simulink model "iddemo_cstr"  (R2016a)
settings: Solver=ode45  StartTime=0  StopTime=800  MaxStep=0.2  RelTol=1e-3
model workspace (MATLAB code in the model file):
  | %Model constants
  | k0                = 34930800;
  | DeltaER       = 5963.6;
  | DeltaH         = -11.92;
  | UA               = 0.3;
  | FV_plus_UA = 1.3;
  | 
  | %Fixed IC
  | Concentration0 = 1.5;
  | FeedCon0         = 10;
  | FeedTemp0       = 295;
  | 
  | %Derived IC
  | tmpVal = FeedCon0/Concentration0-1;
  | ReactorTemp0 = -DeltaER/log(tmpVal/k0);
  | CoolantTemp0 = (ReactorTemp0*(FV_plus_UA)+tmpVal*Concentration0*DeltaH-FeedTemp0)/UA;
  | 
  | %
  | tStep = 400; % [s] When the step reference change happens
  | Ts = 0.1; % [s] Sample time
  | 
  | % Scaling factors on the signals
  | CAscale = 10;
  | Tjscale = 1/10;
  | 
  | % Moving average filter
  | N = 100;
  | 
  | %Clean up
  | clear tmpVal
undefined symbols (not defined in the file or in its folder): sigbuilder_block
libraries: simulink x3, slident x1
settings Model: Creator=The MathWorks, Inc.  LastModifiedBy=The MathWorks, Inc.
settings DataIOCC: InitialState=[311.267; 8.5695]  SaveFormat=Array  SaveOutput=off  SignalLogging=off  DSMLogging=off  SaveTime=off  SignalLoggingName=logsOut
settings OptimizationCC: BlockReduction=off  BooleanDataType=off  DefaultParameterBehavior=Inlined  InlineInvariantSignals=on  BufferReuse=off  ExpressionDepthLimit=2147483647  InitFltsAndDblsToZero=on
settings DebuggingCC: SaveWithParameterizedLinksMsg=none  UnderspecifiedInitializationDetection=Classic  MergeDetectMultiDrivingBlocksExec=none  CheckExecutionContextPreStartOutputMsg=on  CheckExecutionContextRuntimeOutputMsg=on  SignalResolutionControl=TryResolveAllWithWarning  MultiTaskDSMMsg=warning  MultiTaskCondExecSysMsg=none  FcnCallInpInsideContextMsg=UseLocalSettings  AllowSymbolicDim=off  StateNameClashWarn=warning
settings HardwareCC: ProdBitPerPointer=32  ProdLargestAtomicFloat=None  ProdIntDivRoundTo=Undefined  ProdEndianess=Unspecified  ProdWordSize=32  ProdHWDeviceType=32-bit Generic  TargetUnknown=on
settings ModelReferenceCC: PropagateSignalLabelsOutOfModel=off
settings GRTTargetCC: TargetFcnLib=ansi_tfl_tmw.mat  CombineOutputUpdateFcns=off  GRTInterface=on
settings ConfigComp: CovModelRefEnable=Off  CovSFcnEnable=off

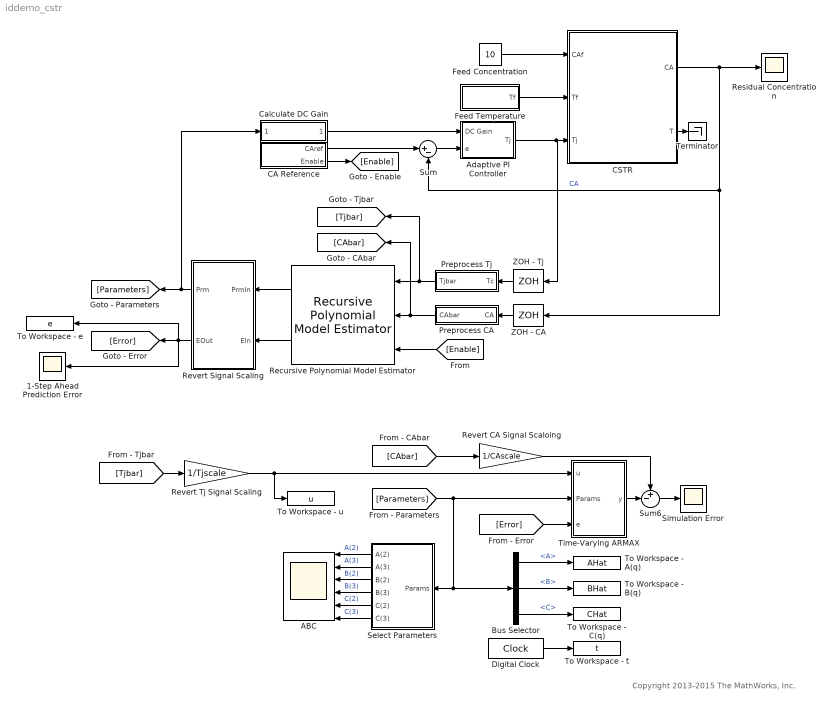
== system iddemo_cstr ==
  note: Copyright 2013-2015 The MathWorks, Inc.
  " Revert CA Signal Scaloing" : Gain  Gain=1/CAscale
  1-Step Ahead Prediction Error : Scope
  ABC : Scope  NumInputPorts=6
  Adaptive PI Controller : Subsystem
  Bus Selector : BusSelector  OutputSignals=A,B,C
  CA Reference : Subsystem
  CSTR : Subsystem
  Calculate DC Gain : Subsystem
  Digital Clock : DigitalClock  SampleTime=Ts
  Feed Concentration : Constant  Value=10
  Feed Temperature : Subsystem
  Preprocess CA : Subsystem
  Preprocess Tj : Subsystem
  Recursive Polynomial Model Estimator : slident/Estimators/Recursive Polynomial Model Estimator  ModelStructure=ARMAX  InitialEstimateSource=None  A0=2  B0=2  C0=2  D0=1  F0=1  nk=1  P0=1e4  EstimationMethod=Forgetting Factor  AdaptationParameter=1-5e-3  NormalizationBias=eps  OutputError=on  OutputP=off  AddEnablePort=on  Ts=0.1
  Residual Concentration : Scope
  Revert Signal Scaling : Subsystem
  Revert Tj Signal Scaling : Gain  Gain=1/Tjscale
  Select Parameters : Subsystem
  Simulation Error : Scope
  Sum : Sum  Inputs=|+-
  Sum6 : Sum  Inputs=+-|
  Terminator : Terminator
  Time-Varying ARMAX : Subsystem
  To Workspace - A(q) : ToWorkspace  VariableName=AHat  SampleTime=-1
  To Workspace - B(q) : ToWorkspace  VariableName=BHat  SampleTime=-1
  To Workspace - C(q) : ToWorkspace  VariableName=CHat  SampleTime=-1
  To Workspace - e : ToWorkspace  VariableName=e  SampleTime=-1
  To Workspace - t : ToWorkspace  VariableName=t  SampleTime=-1
  To Workspace - u : ToWorkspace  VariableName=u  SampleTime=-1
  ZOH - CA : ZeroOrderHold  SampleTime=Ts
  ZOH - Tj : ZeroOrderHold  SampleTime=Ts
  wires:
  CSTR/2(T) -> Terminator/1
  Preprocess Tj/1(Tjbar) -> Recursive Polynomial Model Estimator/1, [Tjbar]
  Preprocess CA/1(CAbar) -> Recursive Polynomial Model Estimator/2, [CAbar]
  Recursive Polynomial Model Estimator/1 -> Revert Signal Scaling/1(PrmIn)
  CSTR/1(CA) -> Residual Concentration/1, ZOH - CA/1, Sum/2  "CA"
  Feed Concentration/1 -> CSTR/1(CAf)
  CA Reference/1(CAref) -> Sum/1
  Feed Temperature/1(Tf) -> CSTR/2(Tf)
  CA Reference/2(Enable) -> [Enable]
  [Enable] -> Recursive Polynomial Model Estimator/3
  Recursive Polynomial Model Estimator/2 -> Revert Signal Scaling/2(EIn)
  Revert Signal Scaling/1(Prm) -> [Parameters], Calculate DC Gain/1(Params)
  ZOH - Tj/1 -> Preprocess Tj/1(Tc)
  ZOH - CA/1 -> Preprocess CA/1(CA)
  Adaptive PI Controller/1(Tj) -> ZOH - Tj/1, CSTR/3(Tj)
  Calculate DC Gain/1(DCGain) -> Adaptive PI Controller/1(DC Gain)
  Sum/1 -> Adaptive PI Controller/2(e)
  Revert Signal Scaling/2(EOut) -> To Workspace - e/1, 1-Step Ahead Prediction Error/1, [Error]
  [Parameters] -> Bus Selector/1, Select Parameters/1(Params), Time-Varying ARMAX/2(Params)
  [Error] -> Time-Varying ARMAX/3(e)
  Bus Selector/1 -> To Workspace - A(q)/1  "<A>"
  Bus Selector/2 -> To Workspace - B(q)/1  "<B>"
  Bus Selector/3 -> To Workspace - C(q)/1  "<C>"
  Revert Tj Signal Scaling/1 -> Time-Varying ARMAX/1(u), To Workspace - u/1
  [Tjbar] -> Revert Tj Signal Scaling/1
  [CAbar] -> " Revert CA Signal Scaloing"/1
  " Revert CA Signal Scaloing"/1 -> Sum6/1
  Time-Varying ARMAX/1(y) -> Sum6/2
  Sum6/1 -> Simulation Error/1
  Select Parameters/4(B(3)) -> ABC/4  "B(3)"
  Select Parameters/3(B(2)) -> ABC/3  "B(2)"
  Select Parameters/5(C(2)) -> ABC/5  "C(2)"
  Select Parameters/2(A(3)) -> ABC/2  "A(3)"
  Select Parameters/6(C(3)) -> ABC/6  "C(3)"
  Select Parameters/1(A(2)) -> ABC/1  "A(2)"
  Digital Clock/1 -> To Workspace - t/1

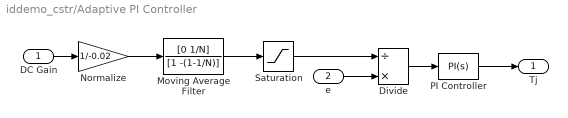
== system iddemo_cstr/Adaptive PI Controller ==
  DC Gain : Inport
  e : Inport  Port=2
  Divide : Product  Inputs=/*
  Moving Average Filter : DiscreteFilter  Numerator=[0 1/N]  Denominator=[1 -(1-1/N)]  InitialStates=N  SampleTime=Ts
  Normalize : Gain  Gain=1/-0.02
  PI Controller : simulink/Continuous/PID Controller  Controller=PI  TimeDomain=Continuous-time  SampleTime=-1  IntegratorMethod=Forward Euler  FilterMethod=Forward Euler  Form=Parallel  UseFilter=on  ControllerParametersSource=internal  P=-13  I=-25  D=0  N=100  InitialConditionSource=internal  InitialConditionForIntegrator=CoolantTemp0  InitialConditionForFilter=0  ExternalReset=none  LimitOutput=off  UpperSaturationLimit=inf  LowerSaturationLimit=-inf  LinearizeAsGain=on  AntiWindupMode=none  Kb=1  TrackingMode=off  Kt=1  PParamMin=[]  PParamMax=[]  IParamMin=[]  IParamMax=[]  DParamMin=[]  DParamMax=[]  NParamMin=[]  NParamMax=[]  KbParamMin=[]  KbParamMax=[]  KtParamMin=[]  KtParamMax=[]  POutMin=[]  POutMax=[]  IOutMin=[]  IOutMax=[]  DOutMin=[]  DOutMax=[]  NOutMin=[]  NOutMax=[]  KbOutMin=[]  KbOutMax=[]  KtOutMin=[]  KtOutMax=[]  IntegratorOutMin=[]  IntegratorOutMax=[]  FilterOutMin=[]  FilterOutMax=[]  SumOutMin=[]  SumOutMax=[]  SumI1OutMin=[]  SumI1OutMax=[]  SumI2OutMin=[]  SumI2OutMax=[]  SumI3OutMin=[]  SumI3OutMax=[]  SumDOutMin=[]  SumDOutMax=[]  SaturationOutMin=[]  SaturationOutMax=[]  IntegratorContinuousStateAttributes=''  IntegratorStateMustResolveToSignalObject=off  IntegratorRTWStateStorageClass=Auto  FilterContinuousStateAttributes=''  FilterStateMustResolveToSignalObject=off  FilterRTWStateStorageClass=Auto  DifferentiatorICPrevScaledInput=0  DifferentiatorOutMin=[]  DifferentiatorOutMax=[]
  Saturation : Saturate  UpperLimit=3  LowerLimit=0.5
  Tj : Outport
  wires:
  e/1 -> Divide/2
  Divide/1 -> PI Controller/1
  PI Controller/1 -> Tj/1
  Moving Average Filter/1 -> Saturation/1
  DC Gain/1 -> Normalize/1
  Normalize/1 -> Moving Average Filter/1
  Saturation/1 -> Divide/1

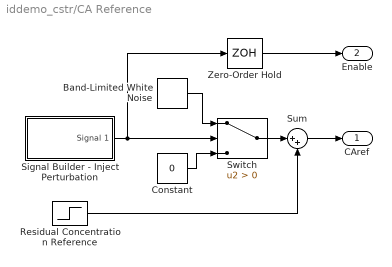
== system iddemo_cstr/CA Reference ==
  Band-Limited White Noise : simulink/Sources/Band-Limited White Noise  Cov=0.015  Ts=Ts  seed=[23341]
  Constant : Constant  Value=0
  Residual Concentration Reference : Step  Time=tStep  Before=Concentration0  After=2  SampleTime=0
  Signal Builder - Inject Perturbation : Subsystem  Tag=STV Subsys  LoadFcn=sigbuilder_block('load');  StartFcn=sigbuilder_block('start');  StopFcn=sigbuilder_block('stop');  ClipboardFcn=sigbuilder_block('clipboard');  mask(Sigbuilder block){}
      mask help: Simulink:masks:SigbuilderBlock_MD
      mask init:
      | if ~strcmp(get_param(bdroot(gcbh),'SimulationStatus'),'stopped') tuvar = sigbuilder_block('maskInit'); end
      settings: CopyFcn=sigbuilder_block('copy');  DeleteFcn=sigbuilder_block('delete');  ModelCloseFcn=sigbuilder_block('modelClose');  PreSaveFcn=sigbuilder_block('preSave');  PauseFcn=sigbuilder_block('pause');  ContinueFcn=sigbuilder_block('continue');  NameChangeFcn=sigbuilder_block('namechange');  OpenFcn=sigbuilder_block('open',[437.25 199.5 550.5 399.75 ]);  CloseFcn=sigbuilder_block('close');
      mask Display: plot(0, 0, 100, 100,[2, 2, 32, 32, 2], [68, 8, 8, 68, 68],[32, 2], [38, 38], [32, 19, 2],[53, 60, 44], [32, 17, 17, 2],[16, 16, 31, 31]);txt = getActiveGroup(gcbh);text(2, 100, txt,'verticalAlignment', 'top');
  Sum : Sum  Inputs=|++
  Switch : Switch  Criteria=u2 > Threshold
  Zero-Order Hold : ZeroOrderHold  SampleTime=Ts
  CAref : Outport
  Enable : Outport  Port=2
  wires:
  Constant/1 -> Switch/3
  Band-Limited White Noise/1 -> Switch/1
  Signal Builder - Inject Perturbation/1(Signal 1) -> Zero-Order Hold/1, Switch/2
  Switch/1 -> Sum/1
  Residual Concentration Reference/1 -> Sum/2
  Sum/1 -> CAref/1
  Zero-Order Hold/1 -> Enable/1

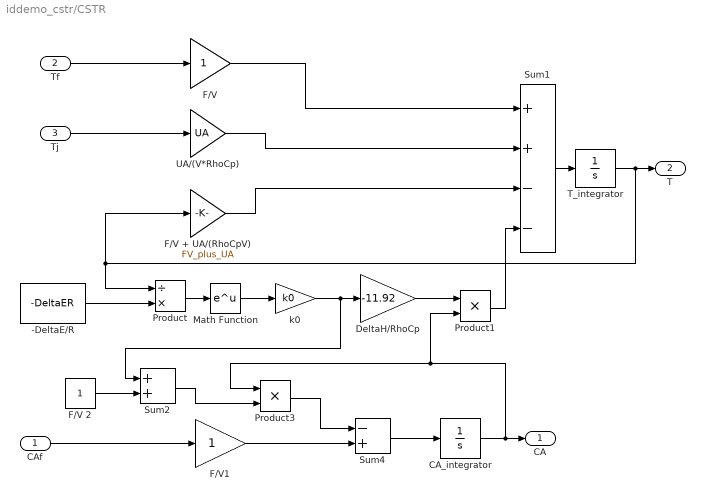
== system iddemo_cstr/CSTR ==
  CAf : Inport
  Tf : Inport  Port=2
  Tj : Inport  Port=3
  -DeltaE/R : Constant  Value=-DeltaER
  CA_integrator : Integrator  InitialCondition=Concentration0  LimitOutput=on  LowerSaturationLimit=0
  DeltaH/RhoCp : Gain  Gain=-11.92  SaturateOnIntegerOverflow=on  OutDataTypeStr=Inherit: Same as input  ParamDataTypeStr=Inherit: Same as input
  F/V : Gain  SaturateOnIntegerOverflow=on  OutDataTypeStr=Inherit: Same as input  ParamDataTypeStr=Inherit: Same as input
  F/V + UA/(RhoCpV) : Gain  Gain=FV_plus_UA  SaturateOnIntegerOverflow=on  OutDataTypeStr=Inherit: Same as input  ParamDataTypeStr=Inherit: Same as input
  F/V 2 : Constant
  F/V1 : Gain  SaturateOnIntegerOverflow=on  OutDataTypeStr=Inherit: Same as input  ParamDataTypeStr=Inherit: Same as input
  Math Function : Math  SaturateOnIntegerOverflow=on
  Product : Product  Inputs=/*  SaturateOnIntegerOverflow=on  RndMeth=Zero  InputSameDT=on  OutDataTypeStr=Inherit: Same as first input
  Product1 : Product  SaturateOnIntegerOverflow=on  RndMeth=Zero  InputSameDT=on  OutDataTypeStr=Inherit: Same as first input
  Product3 : Product  SaturateOnIntegerOverflow=on  RndMeth=Zero  InputSameDT=on  OutDataTypeStr=Inherit: Same as first input
  Sum1 : Sum  Inputs=++--  SaturateOnIntegerOverflow=on  InputSameDT=on  OutDataTypeStr=Inherit: Same as first input
  Sum2 : Sum  SaturateOnIntegerOverflow=on  InputSameDT=on  OutDataTypeStr=Inherit: Same as first input
  Sum4 : Sum  Inputs=-+  SaturateOnIntegerOverflow=on  InputSameDT=on  OutDataTypeStr=Inherit: Same as first input
  T_integrator : Integrator  InitialCondition=ReactorTemp0  LimitOutput=on  LowerSaturationLimit=0
  UA/(V*RhoCp) : Gain  Gain=UA  SaturateOnIntegerOverflow=on  OutDataTypeStr=Inherit: Same as input  ParamDataTypeStr=Inherit: Same as input
  k0 : Gain  Gain=k0  SaturateOnIntegerOverflow=on  OutDataTypeStr=Inherit: Same as input  ParamDataTypeStr=Inherit: Same as input
  CA : Outport
  T : Outport  Port=2
  wires:
  F/V/1 -> Sum1/1
  Sum1/1 -> T_integrator/1
  T_integrator/1 -> Product/1, F/V + UA/(RhoCpV)/1, T/1
  UA/(V*RhoCp)/1 -> Sum1/2
  F/V + UA/(RhoCpV)/1 -> Sum1/3
  Product/1 -> Math Function/1
  Math Function/1 -> k0/1
  DeltaH/RhoCp/1 -> Product1/1
  Product1/1 -> Sum1/4
  k0/1 -> DeltaH/RhoCp/1, Sum2/1
  -DeltaE/R/1 -> Product/2
  Product3/1 -> Sum4/1
  Sum4/1 -> CA_integrator/1
  CA_integrator/1 -> Product1/2, Product3/1, CA/1
  F/V 2/1 -> Sum2/2
  F/V1/1 -> Sum4/2
  Tf/1 -> F/V/1
  CAf/1 -> F/V1/1
  Tj/1 -> UA/(V*RhoCp)/1
  Sum2/1 -> Product3/2

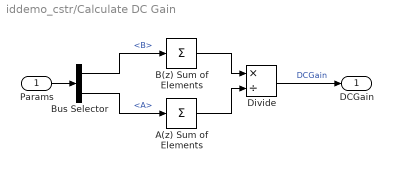
== system iddemo_cstr/Calculate DC Gain ==
  Params : Inport
  A(z) Sum of Elements : Sum  Inputs=+
  B(z) Sum of Elements : Sum  Inputs=+
  Bus Selector : BusSelector  OutputSignals=B,A
  Divide : Product  Inputs=*/
  DCGain : Outport
  wires:
  A(z) Sum of Elements/1 -> Divide/2
  B(z) Sum of Elements/1 -> Divide/1
  Params/1 -> Bus Selector/1
  Bus Selector/1 -> B(z) Sum of Elements/1  "<B>"
  Bus Selector/2 -> A(z) Sum of Elements/1  "<A>"
  Divide/1 -> DCGain/1  "DCGain"

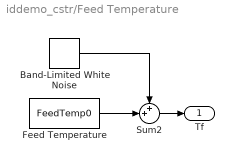
== system iddemo_cstr/Feed Temperature ==
  Band-Limited White Noise : simulink/Sources/Band-Limited White Noise  Cov=0.0075  Ts=Ts  seed=[23341]
  Feed Temperature : Constant  Value=FeedTemp0
  Sum2 : Sum  Inputs=++|
  Tf : Outport
  wires:
  Band-Limited White Noise/1 -> Sum2/1
  Feed Temperature/1 -> Sum2/2
  Sum2/1 -> Tf/1

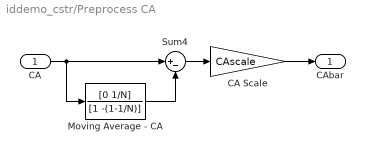
== system iddemo_cstr/Preprocess CA ==
  CA : Inport
  CA Scale : Gain  Gain=CAscale
  Moving Average - CA : DiscreteFilter  Numerator=[0 1/N]  Denominator=[1 -(1-1/N)]  InitialStates=Concentration0*N  SampleTime=Ts
  Sum4 : Sum  Inputs=|+-
  CAbar : Outport
  wires:
  CA/1 -> Moving Average - CA/1, Sum4/1
  Moving Average - CA/1 -> Sum4/2
  Sum4/1 -> CA Scale/1
  CA Scale/1 -> CAbar/1

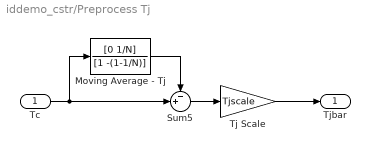
== system iddemo_cstr/Preprocess Tj ==
  Tc : Inport
  Moving Average - Tj : DiscreteFilter  Numerator=[0 1/N]  Denominator=[1 -(1-1/N)]  InitialStates=CoolantTemp0*N  SampleTime=Ts
  Sum5 : Sum  Inputs=-+|
  Tj Scale : Gain  Gain=Tjscale
  Tjbar : Outport
  wires:
  Tc/1 -> Moving Average - Tj/1, Sum5/2
  Moving Average - Tj/1 -> Sum5/1
  Sum5/1 -> Tj Scale/1
  Tj Scale/1 -> Tjbar/1

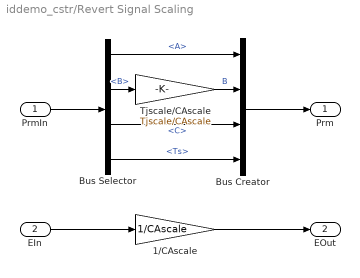
== system iddemo_cstr/Revert Signal Scaling ==
  PrmIn : Inport
  EIn : Inport  Port=2
  1/CAscale : Gain  Gain=1/CAscale
  Bus Creator : BusCreator  Inputs=4
  Bus Selector : BusSelector  OutputSignals=A,B,C,Ts
  Tjscale/CAscale : Gain  Gain=Tjscale/CAscale
  Prm : Outport
  EOut : Outport  Port=2
  wires:
  EIn/1 -> 1/CAscale/1
  PrmIn/1 -> Bus Selector/1
  Bus Selector/1 -> Bus Creator/1  "<A>"
  Bus Selector/4 -> Bus Creator/4  "<Ts>"
  Bus Selector/3 -> Bus Creator/3  "<C>"
  Bus Selector/2 -> Tjscale/CAscale/1  "<B>"
  Tjscale/CAscale/1 -> Bus Creator/2  "B"
  1/CAscale/1 -> EOut/1
  Bus Creator/1 -> Prm/1

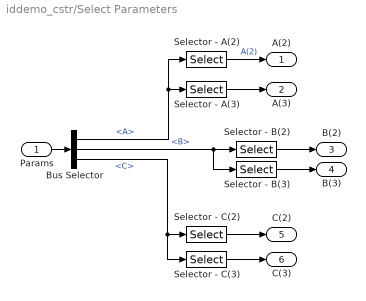
== system iddemo_cstr/Select Parameters ==
  Params : Inport
  Bus Selector : BusSelector  OutputSignals=A,B,C
  Selector - A(2) : Selector  NumberOfDimensions=2  InputPortWidth=3  IndexOptions=Index vector (dialog),Index vector (dialog)  Indices=1,2  OutputSizes=1,1
  Selector - A(3) : Selector  NumberOfDimensions=2  InputPortWidth=3  IndexOptions=Index vector (dialog),Index vector (dialog)  Indices=1,3  OutputSizes=1,1
  Selector - B(2) : Selector  NumberOfDimensions=2  InputPortWidth=3  IndexOptions=Index vector (dialog),Index vector (dialog)  Indices=1,2  OutputSizes=1,1
  Selector - B(3) : Selector  NumberOfDimensions=2  InputPortWidth=3  IndexOptions=Index vector (dialog),Index vector (dialog)  Indices=1,3  OutputSizes=1,1
  Selector - C(2) : Selector  NumberOfDimensions=2  InputPortWidth=3  IndexOptions=Index vector (dialog),Index vector (dialog)  Indices=1,2  OutputSizes=1,1
  Selector - C(3) : Selector  NumberOfDimensions=2  InputPortWidth=3  IndexOptions=Index vector (dialog),Index vector (dialog)  Indices=1,3  OutputSizes=1,1
  A(2) : Outport
  A(3) : Outport  Port=2
  B(2) : Outport  Port=3
  B(3) : Outport  Port=4
  C(2) : Outport  Port=5
  C(3) : Outport  Port=6
  wires:
  Params/1 -> Bus Selector/1
  Bus Selector/1 -> Selector - A(2)/1, Selector - A(3)/1  "<A>"
  Bus Selector/2 -> Selector - B(3)/1, Selector - B(2)/1  "<B>"
  Bus Selector/3 -> Selector - C(3)/1, Selector - C(2)/1  "<C>"
  Selector - A(3)/1 -> A(3)/1
  Selector - A(2)/1 -> A(2)/1  "A(2)"
  Selector - B(2)/1 -> B(2)/1
  Selector - B(3)/1 -> B(3)/1
  Selector - C(2)/1 -> C(2)/1
  Selector - C(3)/1 -> C(3)/1

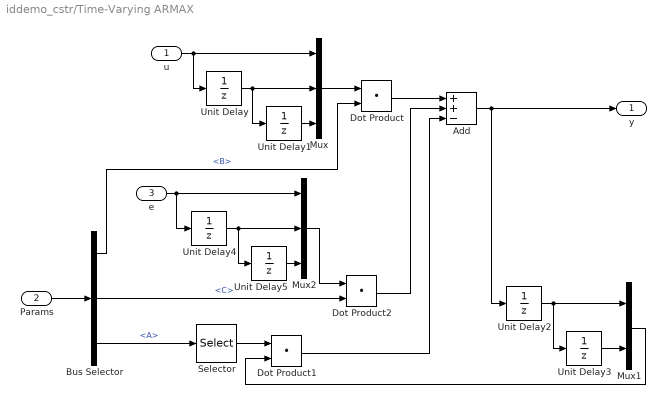
== system iddemo_cstr/Time-Varying ARMAX ==
  u : Inport
  Params : Inport  Port=2
  e : Inport  Port=3
  Add : Sum  Inputs=++-
  Bus Selector : BusSelector  OutputSignals=B,C,A
  Dot Product : DotProduct  InputSameDT=on  OutDataTypeStr=Inherit: Inherit via internal rule
  Dot Product1 : DotProduct  InputSameDT=on  OutDataTypeStr=Inherit: Inherit via internal rule
  Dot Product2 : DotProduct  InputSameDT=on  OutDataTypeStr=Inherit: Inherit via internal rule
  Mux : Mux  Inputs=3
  Mux1 : Mux  Inputs=2
  Mux2 : Mux  Inputs=3
  Selector : Selector  NumberOfDimensions=2  InputPortWidth=3  IndexOptions=Index vector (dialog),Index vector (dialog)  Indices=1,[2 3]  OutputSizes=1,1
  Unit Delay{,1..5} (6 alike) : UnitDelay  SampleTime=-1
  y : Outport
  wires:
  Unit Delay/1 -> Unit Delay1/1, Mux/2
  Mux/1 -> Dot Product/1
  Bus Selector/1 -> Dot Product/2  "<B>"
  Unit Delay1/1 -> Mux/3
  u/1 -> Unit Delay/1, Mux/1
  Bus Selector/3 -> Selector/1  "<A>"
  Add/1 -> y/1, Unit Delay2/1
  Unit Delay2/1 -> Unit Delay3/1, Mux1/1
  Dot Product/1 -> Add/1
  Unit Delay3/1 -> Mux1/2
  Selector/1 -> Dot Product1/1
  e/1 -> Unit Delay4/1, Mux2/1
  Bus Selector/2 -> Dot Product2/2  "<C>"
  Dot Product1/1 -> Add/3
  Mux1/1 -> Dot Product1/2
  Dot Product2/1 -> Add/2
  Params/1 -> Bus Selector/1
  Unit Delay4/1 -> Unit Delay5/1, Mux2/2
  Unit Delay5/1 -> Mux2/3
  Mux2/1 -> Dot Product2/1

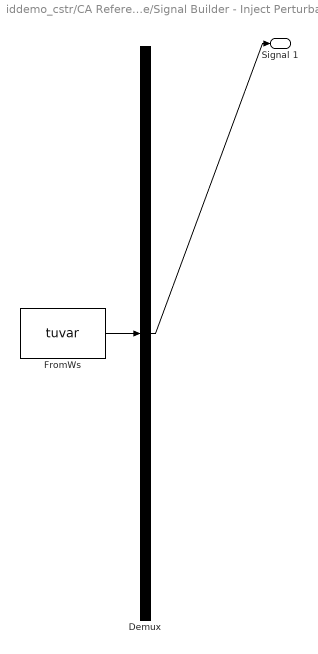
== system iddemo_cstr/CA Reference/Signal Builder - Inject Perturbation ==
  Demux : Demux  Tag=STV Demux  Outputs=1
  FromWs : FromWorkspace  Tag=STV FromWs  VariableName=tuvar  SampleTime=0
      SigBuilderData=|
      | common.afterFinalStr = 'Extrapolate'
      | common.sampleTime = 0
      | dataSet(1).timeRange = [0 1800]
      | dataSet(1).name = 'Group 1'
      | dataSet(2).timeRange = [0 1200]
      | dataSet(2).name = 'Group 2'
      | sbobj.Groups(1).Name = 'Group 1'
      | sbobj.Groups(1).Signals.Name = 'Signal 1'
      | sbobj.Groups(1).Signals.XData = [0 200 200 1800]
      | sbobj.Groups(1).Signals.YData = [1 1 0 0]
      | sbobj.Groups(1).TimeRange = [0 1800]
      | sbobj.Groups(2).Name = 'Group 2'
      | sbobj.Groups(2).Signals.Name = 'Signal 1'
      | sbobj.Groups(2).Signals.XData = [0 198 198 400 400 600 600 1200]
      | sbobj.Groups(2).Signals.YData = [1 1 0 0 1 1 0 0]
      | sbobj.Groups(2).TimeRange = [0 1200]
  Signal 1 : Outport  Tag=STV Outport
  wires:
  FromWs/1 -> Demux/1
  Demux/1 -> Signal 1/1
